simulink model "limit_test_function_211218"  (R2018b)
settings: Solver=FixedStepAuto  StartTime=0.0  StopTime=10.0  FixedStep=0.001  RelTol=1e-3
settings Model: Creator=Paweł Tymiński  LastModifiedBy=Paweł Tymiński

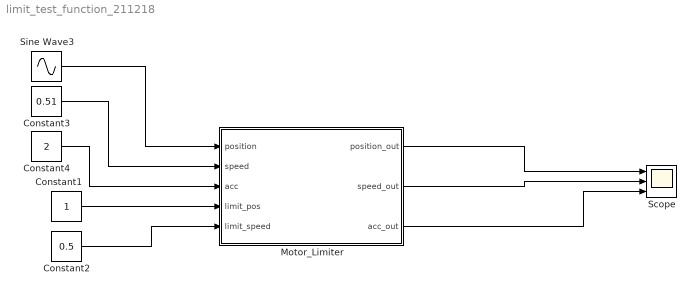
== system limit_test_function_211218 ==
  Constant1 : Constant
  Constant2 : Constant  Value=0.5
  Constant3 : Constant  Value=0.51
  Constant4 : Constant  Value=2
  Motor_Limiter : MATLAB Function  TreatAsAtomicUnit=on
  Scope : Scope  NumInputPorts=3
  Sine Wave3 : Sin  Amplitude=1.5  SampleTime=0
  wires:
  Sine Wave3/1 -> Motor_Limiter/1(position)
  Constant1/1 -> Motor_Limiter/4(limit_pos)
  Motor_Limiter/1(position_out) -> Scope/1
  Constant3/1 -> Motor_Limiter/2(speed)
  Constant2/1 -> Motor_Limiter/5(limit_speed)
  Motor_Limiter/2(speed_out) -> Scope/2
  Constant4/1 -> Motor_Limiter/3(acc)
  Motor_Limiter/3(acc_out) -> Scope/3

== matlab function limit_test_function_211218/Motor_Limiter ==
  data: position input; position_out output; speed input; speed_out output; acc input; limit_pos input; limit_speed input; acc_out output
function [position_out,speed_out,acc_out] = fcn(position, speed,  acc, limit_pos, limit_speed)
if abs(position)>=limit_pos  & abs(speed) >= limit_speed
	position_out=sign(position)*limit_pos;
	speed_out=0;
	acc_out=0;
elseif abs(position)>=limit_pos  & abs(speed) <= limit_speed
	position_out=sign(position)*limit_pos;
	speed_out=0;
	acc_out=0;	
elseif	abs(position)<=limit_pos  & abs(speed) >= limit_speed
	position_out=position;
	speed_out=sign(speed)*limit_speed;
	acc_out=0;	
else 	
    position_out=position;
    speed_out=speed;
    acc_out=acc;
end
